simulink model "massignment1"  (Simulink 6.0)
settings: Solver=FixedStepDiscrete  StartTime=0.0  StopTime=10.0  RelTol=1e-3
settings Model: Creator=awarlock  LastModifiedBy=awarlock  ExtModeAutoUpdateStatusClock=off
settings OptimizationCC: InlineParams=on
settings DebuggingCC: MultiTaskDSMMsg=warning

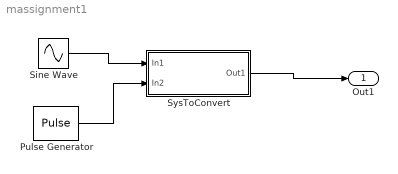
== system massignment1 ==
  Pulse Generator : DiscretePulseGenerator  SampleTime=0.1
  Sine Wave : Sin  Amplitude=3:7  SampleTime=0.1
  SysToConvert : Subsystem  TreatAsAtomicUnit=on
  Out1 : Outport
  wires:
  Sine Wave/1 -> SysToConvert/1(In1)
  Pulse Generator/1 -> SysToConvert/2(In2)
  SysToConvert/1(Out1) -> Out1/1

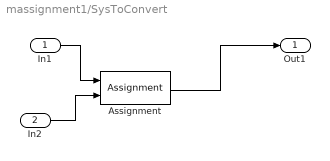
== system massignment1/SysToConvert ==
  In1 : Inport  Port=1  LatchInput=off
  In2 : Inport  Port=2  LatchInput=off
  Assignment : Assignment
  Out1 : Outport
  wires:
  In1/1 -> Assignment/1
  In2/1 -> Assignment/2
  Assignment/1 -> Out1/1
